simulink model "montage1"  (Simulink 7.5)
settings: Solver=ode45  StartTime=0.0  StopTime=Tsim  RelTol=1e-3
values from neighbouring files (symbols this model uses):
  Te = 1/Fe    (= 3.125e-06)    [Bode_partie1.m]    (also in fft_script.m = 0.03125; script.m = 0.03125; script1.m; script2.m)
settings Model: Creator=abdala  LastModifiedBy=Yann
settings DebuggingCC: FcnCallInpInsideContextMsg=Enable All
settings GRTTargetCC: CombineOutputUpdateFcns=on

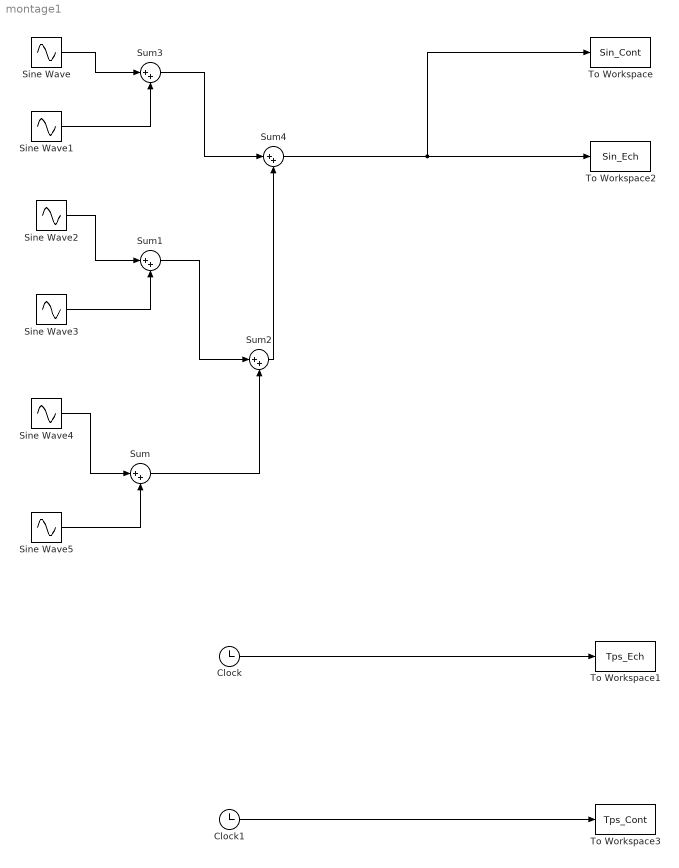
== system montage1 ==
  Clock : Clock
      settings: Decimation=100
  Clock1 : Clock
      settings: Decimation=10
  Sine Wave : Sin  Amplitude=1  Bias=0  Frequency=85000 *2*pi  Phase=0  Samples=10  SampleTime=0  Offset=0
  Sine Wave1 : Sin  Amplitude=1  Bias=0  Frequency=90000*2*pi  Phase=0  Samples=10  SampleTime=0  Offset=0
  Sine Wave2 : Sin  Amplitude=1  Bias=0  Frequency=95000*2*pi  Phase=0  Samples=10  SampleTime=0  Offset=0
  Sine Wave3 : Sin  Amplitude=1  Bias=0  Frequency=100000*2*pi  Phase=0  Samples=10  SampleTime=0  Offset=0
  Sine Wave4 : Sin  Amplitude=1  Bias=0  Frequency=115000*2*pi  Phase=0  Samples=10  SampleTime=0  Offset=0
  Sine Wave5 : Sin  Amplitude=1  Bias=0  Frequency=120000*2*pi  Phase=0  Samples=10  SampleTime=0  Offset=0
  Sum{,1..4} (5 alike) : Sum  Inputs=|++
  To Workspace : ToWorkspace  VariableName=Sin_Cont  SampleTime=Te/100  SaveFormat=Array
  To Workspace1 : ToWorkspace  VariableName=Tps_Ech  SampleTime=Te  SaveFormat=Array
  To Workspace2 : ToWorkspace  VariableName=Sin_Ech  SampleTime=Te  SaveFormat=Array
  To Workspace3 : ToWorkspace  VariableName=Tps_Cont  SampleTime=Te/100  SaveFormat=Array
  wires:
  Clock/1 -> To Workspace1/1
  Clock1/1 -> To Workspace3/1
  Sine Wave4/1 -> Sum/1
  Sine Wave5/1 -> Sum/2
  Sine Wave2/1 -> Sum1/1
  Sine Wave3/1 -> Sum1/2
  Sum/1 -> Sum2/2
  Sum1/1 -> Sum2/1
  Sine Wave/1 -> Sum3/1
  Sine Wave1/1 -> Sum3/2
  Sum3/1 -> Sum4/1
  Sum2/1 -> Sum4/2
  Sum4/1 -> To Workspace2/1, To Workspace/1
